simulink model "problem8"  (R2020a)
settings: Solver=VariableStepAuto  StartTime=0.0  StopTime=10.0  RelTol=1e-3
undefined symbols (not defined in the file): sigbuilder_block
libraries: simulink x2
settings Model: EnablePacing=on  PacingRate=0.220000  Creator=Jake  LastModifiedBy=Jake

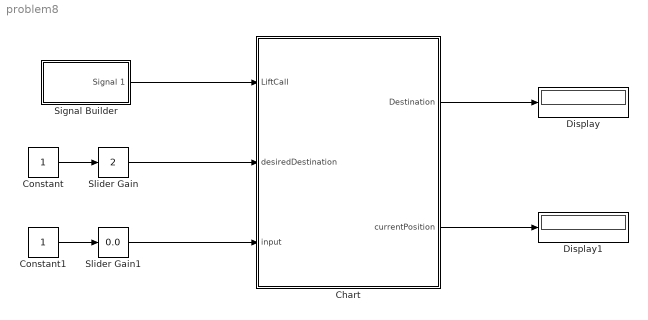
== system problem8 ==
  Chart : Stateflow chart  TreatAsAtomicUnit=on
  Constant : Constant
  Constant1 : Constant
  Display : Display
  Display1 : Display
  Signal Builder : Subsystem  Tag=STV Subsys  LoadFcn=sigbuilder_block('load');  StartFcn=sigbuilder_block('start');  StopFcn=sigbuilder_block('stop');  ClipboardFcn=sigbuilder_block('clipboard');  mask(Sigbuilder block){tuvar=[0:10]}
      mask help: Simulink:masks:SigbuilderBlock_MD
      mask init:
      | if ~strcmp(get_param(bdroot(gcbh),'SimulationStatus'),'stopped') tuvar = sigbuilder_block('maskInit'); end
      settings: CopyFcn=sigbuilder_block('copy');  DeleteFcn=sigbuilder_block('delete');  ModelCloseFcn=sigbuilder_block('modelClose');  PreSaveFcn=sigbuilder_block('preSave');  PauseFcn=sigbuilder_block('pause');  ContinueFcn=sigbuilder_block('continue');  NameChangeFcn=sigbuilder_block('namechange');  OpenFcn=sigbuilder_block('open',[404 117.5 550.5 362.5 ]);  CloseFcn=sigbuilder_block('close');
      mask Display: plot(0, 0, 100, 100,[2, 2, 32, 32, 2], [68, 8, 8, 68, 68],[32, 2], [38, 38], [32, 19, 2],[53, 60, 44], [32, 17, 17, 2],[16, 16, 31, 31]);txt = getActiveGroup(gcbh);text(2, 100, txt,'verticalAlignment', 'top');
  Slider Gain : simulink/Math Operations/Slider Gain  gain=2  low=0  high=4
  Slider Gain1 : simulink/Math Operations/Slider Gain  gain=0.0  low=0  high=4
  wires:
  Signal Builder/1(Signal 1) -> Chart/1(LiftCall)
  Constant/1 -> Slider Gain/1
  Slider Gain/1 -> Chart/2(desiredDestination)
  Slider Gain1/1 -> Chart/3(input)
  Constant1/1 -> Slider Gain1/1
  Chart/1(Destination) -> Display/1
  Chart/2(currentPosition) -> Display1/1

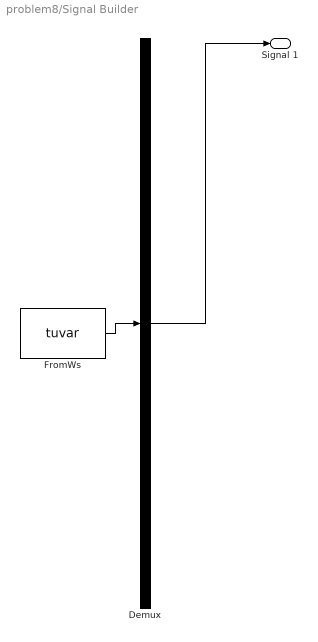
== system problem8/Signal Builder ==
  Demux : Demux  Tag=STV Demux  Outputs=1
      settings: DisplayOption=none
  FromWs : FromWorkspace  Tag=STV FromWs  VariableName=tuvar
      SigBuilderData=|
      | common.afterFinalStr = 'Extrapolate'
      | common.sampleTime = 0
      | dataSet.timeRange = [0 10]
      | dataSet.name = 'Group 1'
      | sbobj.Groups.Name = 'Group 1'
      | sbobj.Groups.Signals.Name = 'Signal 1'
      | sbobj.Groups.Signals.XData = [0 2.98 2.98 3.68 3.68 10]
      | sbobj.Groups.Signals.YData = [0 0 1 1 -0.005 0]
  Signal 1 : Outport  Tag=STV Outport
  wires:
  Demux/1 -> Signal 1/1
  FromWs/1 -> Demux/1

== stateflow chart problem8/Chart ==
  state Stopped
    state stoppedAndWaiting
      state intialise
        entry: motor=false;
        brakeoff=false;
        doors=false;
        Destinationreached= false;
        commandprocessing=false;
      state settingdown
        entry:
        up=false;
      state destination
        Destination=desiredDestination;
        currentPosition=input;
      state settingup
        entry:
        up=true;
      state commandDone
        commandprocessing=true;
      (default) -> intialise
      intialise -> intialise [order 2] : [~LiftCall&&~commandprocessing]
      intialise -> destination [order 1] : [LiftCall]
      destination -> settingdown [order 2] : [currentPosition>desiredDestination]
      destination -> settingup [order 1] : [currentPosition<desiredDestination]
      settingdown -> commandDone
      settingup -> commandDone
    state stopAtDestination
      state stopLift
        entry:
        motor=false;
        brakeoff=false;
      state ErrorState
        entry:
        doors=false;
      state Openingdoors
        entry:
        Destinationreached=true;
        doors=true;
      (default) -> stopLift
      stopLift -> ErrorState [order 2] : [~currentPosition==desiredDestination]
      stopLift -> Openingdoors [order 1] : [currentPosition==desiredDestination]
    (default) -> stoppedAndWaiting
    stopAtDestination -> stoppedAndWaiting : [doors]
    destination -> stopAtDestination [order 3] : [currentPosition==desiredDestination]
  state Moving
    state startingmotor
      entry:
      motor=true;
      brakeoff=true;
      doors=false;
    state Movingup
      entry:
      currentPosition = currentPosition + 1;
    state Movingdown
      entry:
      currentPosition = currentPosition - 1;
    Movingdown -> Movingdown : [currentPosition>desiredDestination]
    (default) -> startingmotor
    startingmotor -> Movingdown [order 2] : [~up]
    Movingup -> Movingup : [currentPosition<desiredDestination]
    startingmotor -> Movingup [order 1] : [up]
  (default) -> Stopped
  Moving -> stopAtDestination : [currentPosition==desiredDestination]
  stoppedAndWaiting -> Moving : [commandprocessing]
  data: LiftCall input; desiredDestination input; commandprocessing local; up local; input input; brakeoff local; motor local; Destination output; currentPosition output; doors local; Destinationreached local
